simulink model "lab5"  (R2022b)
settings: Solver=VariableStepAuto  StartTime=0.0  StopTime=10.0  RelTol=1e-3
values from neighbouring files (symbols this model uses):
  k1 = 54700    [lab5_dane.m]
  k2 = 303600    [lab5_dane.m]
  m1 = 14000    [lab5_dane.m]
  m2 = 450.28    [lab5_dane.m]
  m3 = 200    [lab5_dane.m]
settings Model: Creator=karol  LastModifiedBy=karol

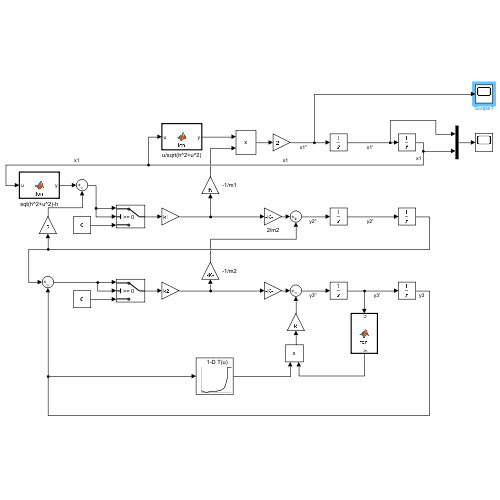
[thumbnail: Simulink's stored preview of the top-level diagram]
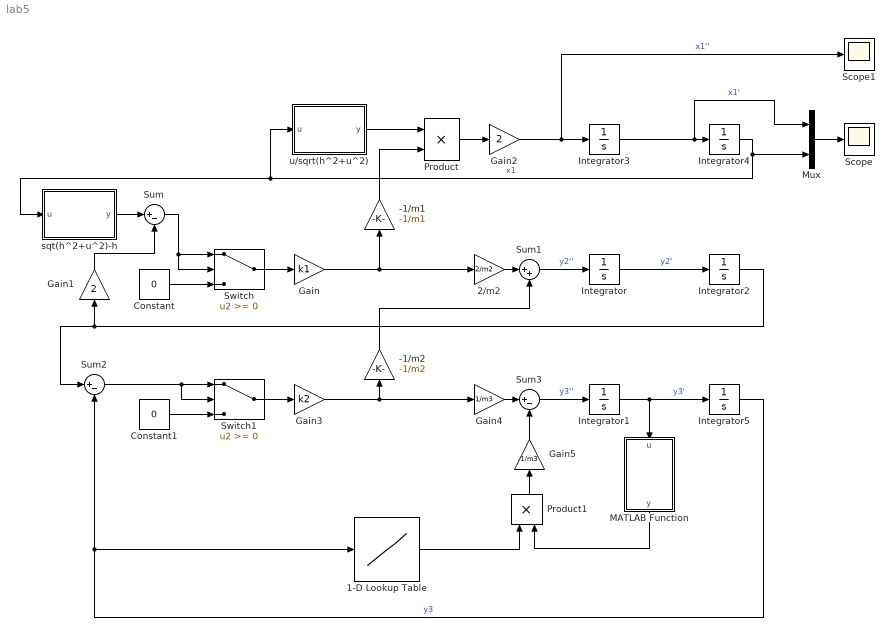
== system lab5 ==
  -1/m1 : Gain  Gain=-1/m1
  -1/m2 : Gain  Gain=-1/m2
  1-D Lookup Table : Lookup_n-D  NumberOfTableDimensions=1  BreakpointsForDimension1=[0, 10, 20, 30, 40, 50, 60, 70, 80, 90, 94, 98, 102, 104, 107, 120]  Table=[833, 400, 160, 320, 520, 520, 660, 830, 1070, 1600, 2100, 2800, 4100, 5000, 9000, 9000]  InternalRulePriority=Speed  RndMeth=Simplest
  2/m2 : Gain  Gain=2/m2
  Constant : Constant  Value=0
  Constant1 : Constant  Value=0
  Gain : Gain  Gain=k1
  Gain1 : Gain  Gain=2
  Gain2 : Gain  Gain=2
  Gain3 : Gain  Gain=k2
  Gain4 : Gain  Gain=1/m3
  Gain5 : Gain  Gain=1/m3
  Integrator{,1..2,4..5} (5 alike) : Integrator
  Integrator3 : Integrator  InitialCondition=67
  MATLAB Function : MATLAB Function  TreatAsAtomicUnit=on
  Mux : Mux  Inputs=2
  Product : Product
  Product1 : Product
  Scope : Scope
  Scope1 : Scope
  Sum : Sum  Inputs=|+-
  Sum1 : Sum  Inputs=|++
  Sum2 : Sum  Inputs=|+-
  Sum3 : Sum  Inputs=|+-
  Switch : Switch  SaturateOnIntegerOverflow=off  InputSameDT=off
  Switch1 : Switch  SaturateOnIntegerOverflow=off  InputSameDT=off
  sqt(h^2+u^2)-h : MATLAB Function  TreatAsAtomicUnit=on
  u/sqrt(h^2+u^2) : MATLAB Function  TreatAsAtomicUnit=on
  wires:
  Constant/1 -> Switch/3
  Switch/1 -> Gain/1
  sqt(h^2+u^2)-h/1(y) -> Sum/1
  Gain1/1 -> Sum/2
  Sum/1 -> Switch/2, Switch/1
  Gain/1 -> -1/m1/1, 2/m2/1
  2/m2/1 -> Sum1/1
  Sum1/1 -> Integrator/1  "y2''"
  Integrator/1 -> Integrator2/1  "y2'"
  Integrator2/1 -> Sum2/1, Gain1/1
  Product/1 -> Gain2/1
  -1/m1/1 -> Product/2
  u/sqrt(h^2+u^2)/1(y) -> Product/1
  Gain2/1 -> Scope1/1, Integrator3/1  "x1''"
  Integrator3/1 -> Mux/1, Integrator4/1  "x1'"
  Mux/1 -> Scope/1
  Integrator4/1 -> Mux/2, sqt(h^2+u^2)-h/1(u), u/sqrt(h^2+u^2)/1(u)  "x1"
  Sum2/1 -> Switch1/2, Switch1/1
  Constant1/1 -> Switch1/3
  Switch1/1 -> Gain3/1
  Gain3/1 -> Gain4/1, -1/m2/1
  Gain4/1 -> Sum3/1
  Sum3/1 -> Integrator1/1  "y3''"
  Integrator1/1 -> Integrator5/1, MATLAB Function/1(u)  "y3'"
  Integrator5/1 -> Sum2/2, 1-D Lookup Table/1  "y3"
  Product1/1 -> Gain5/1
  Gain5/1 -> Sum3/2
  1-D Lookup Table/1 -> Product1/1
  -1/m2/1 -> Sum1/2
  MATLAB Function/1(y) -> Product1/2

== matlab function lab5/u//sqrt(h^2+u^2) ==
  data: u input; y output
function y = fcn(u)
h = 42
y = u/sqrt(u^2 + h^2);

== matlab function lab5/MATLAB Function ==
  data: u input; y output
function y = fcn(u)

y = u^2;

== matlab function lab5/sqt(h^2+u^2)-h ==
  data: u input; y output
function y = fcn(u)
h = 42
y = sqrt(h^2+u^2)-h;
